simulink model "IIR_TF_I"  (Simulink 6.5)
settings: Solver=FixedStepDiscrete  StartTime=0.0  StopTime=16/1000000  RelTol=1e-3
settings Model: Creator=shahein  LastModifiedBy=shahein  ExtModeAutoUpdateStatusClock=off

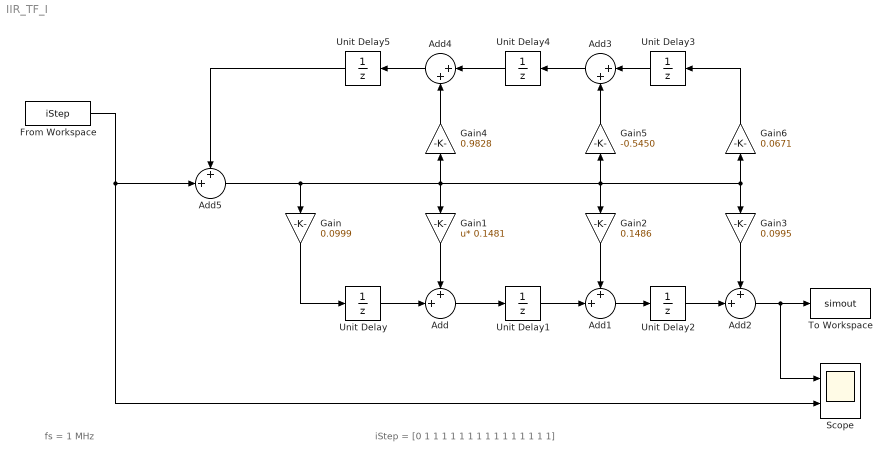
== system IIR_TF_I ==
  note: fs = 1 MHz
  note: iStep = [0 1 1 1 1 1 1 1 1 1 1 1 1 1 1 1]
  Add{,1..2,5} (4 alike) : Sum  Inputs=++|  OutScaling=2^-10
  Add3 : Sum  Orientation=left  Inputs=|++  OutScaling=2^-10
  Add4 : Sum  Orientation=left  Inputs=|++  OutScaling=2^-10
  From Workspace : FromWorkspace  VariableName=iStep  SampleTime=1/1000000  Interpolate=off  OutputAfterFinalValue=Holding final value
  Gain : Gain  Orientation=down  Gain=0.0999
  Gain1 : Gain  Orientation=down  Gain=0.1481  Multiplication=Matrix(u*K)
  Gain2 : Gain  Orientation=down  Gain=0.1486
  Gain3 : Gain  Orientation=down  Gain=0.0995
  Gain4 : Gain  Orientation=up  Gain=0.9828
  Gain5 : Gain  Orientation=up  Gain=-0.5450
  Gain6 : Gain  Orientation=up  Gain=0.0671
  Scope : Scope  NumInputPorts=2
      settings: TimeRange=1.6e-05  YMin=-5~-5  YMax=5~5
  To Workspace : ToWorkspace  VariableName=simout  SampleTime=-1  SaveFormat=Structure
  Unit Delay : UnitDelay  SampleTime=1/1000000
  Unit Delay1 : UnitDelay  SampleTime=1/1000000
  Unit Delay2 : UnitDelay  SampleTime=1/1000000
  Unit Delay3 : UnitDelay  Orientation=left  SampleTime=1/1000000
  Unit Delay4 : UnitDelay  Orientation=left  SampleTime=1/1000000
  Unit Delay5 : UnitDelay  Orientation=left  SampleTime=1/1000000
  wires:
  Gain/1 -> Unit Delay/1
  Gain1/1 -> Add/1
  Gain2/1 -> Add1/1
  Gain3/1 -> Add2/1
  Unit Delay/1 -> Add/2
  Add/1 -> Unit Delay1/1
  Unit Delay1/1 -> Add1/2
  Add1/1 -> Unit Delay2/1
  Unit Delay2/1 -> Add2/2
  Gain6/1 -> Unit Delay3/1
  Unit Delay3/1 -> Add3/1
  Gain5/1 -> Add3/2
  Add3/1 -> Unit Delay4/1
  Unit Delay4/1 -> Add4/1
  Add4/1 -> Unit Delay5/1
  Gain4/1 -> Add4/2
  Unit Delay5/1 -> Add5/1
  Add5/1 -> Gain6/1, Gain3/1, Gain2/1, Gain5/1, Gain1/1, Gain4/1, Gain/1
  Add2/1 -> To Workspace/1, Scope/1
  From Workspace/1 -> Add5/2, Scope/2
